simulink model "invpend_NL_lead"  (R2023b)
settings: Solver=VariableStepAuto  StartTime=0.0  StopTime=10.0  MaxStep=0.01  RelTol=1e-3
settings Model: Creator=bwang-ccny  LastModifiedBy=bwang-ccny

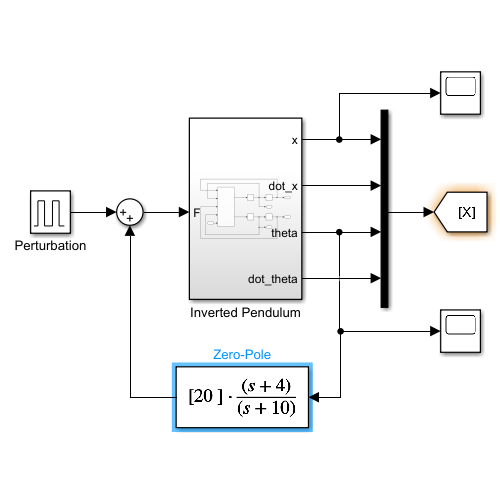
[thumbnail: Simulink's stored preview of the top-level diagram]
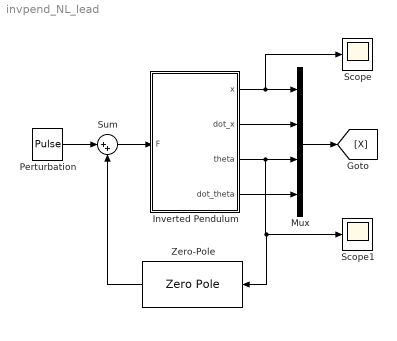
== system invpend_NL_lead ==
  Inverted Pendulum : Subsystem
  Mux : Mux
  Perturbation : DiscretePulseGenerator  PulseType=Time based  Amplitude=10  Period=100  PulseWidth=0.1
  Scope : Scope
  Scope1 : Scope
  Sum : Sum  Inputs=|++
  Zero-Pole : ZeroPole  Zeros=[-4]  Poles=[-10]  Gain=[20]
  wires:
  Inverted Pendulum/1(x) -> Scope/1, Mux/1
  Inverted Pendulum/2(dot_x) -> Mux/2
  Inverted Pendulum/3(theta) -> Zero-Pole/1, Scope1/1, Mux/3
  Inverted Pendulum/4(dot_theta) -> Mux/4
  Mux/1 -> [X]
  Sum/1 -> Inverted Pendulum/1(F)
  Perturbation/1 -> Sum/1
  Zero-Pole/1 -> Sum/2

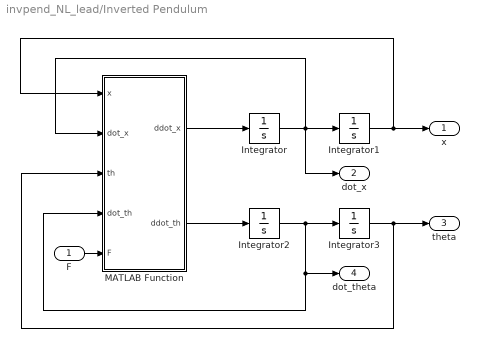
== system invpend_NL_lead/Inverted Pendulum ==
  F : Inport
  Integrator{,1..3} (4 alike) : Integrator
  MATLAB Function : MATLAB Function  TreatAsAtomicUnit=on
  x : Outport
  dot_x : Outport  Port=2
  theta : Outport  Port=3
  dot_theta : Outport  Port=4
  wires:
  Integrator/1 -> dot_x/1, MATLAB Function/2(dot_x), Integrator1/1
  MATLAB Function/2(ddot_th) -> Integrator2/1
  Integrator2/1 -> dot_theta/1, MATLAB Function/4(dot_th), Integrator3/1
  Integrator1/1 -> x/1, MATLAB Function/1(x)
  Integrator3/1 -> theta/1, MATLAB Function/3(th)
  MATLAB Function/1(ddot_x) -> Integrator/1
  F/1 -> MATLAB Function/5(F)

== matlab function invpend_NL_lead/Inverted Pendulum/MATLAB Function ==
  data: x input; ddot_x output; dot_x input; th input; dot_th input; ddot_th output; F input
function [ddot_x, ddot_th] = fcn(x,dot_x,th,dot_th,F)

M = 0.5;
m = 0.2;
I = 0.006;
g = 9.8;
l = 0.3;
Q = (M + m)*(I + m*l^2) - (m*l)^2*cos(th)^2;


ddot_x = ((I + m*l^2)*(F + m*l*dot_th^2*sin(th)) - m^2*l^2*g*cos(th)*sin(th))/Q;
ddot_th = (m*l*cos(th)*F + m^2*l^2*dot_th^2*sin(th)*cos(th) - (M + m)*m*l*g*sin(th))/(-Q);
